simulink model "engine_model"  (R2023b)
settings: Solver=VariableStepAuto  StartTime=0.0  StopTime=10.0  RelTol=1e-3
settings Model: Creator=kirill  LastModifiedBy=kirill
settings DebuggingCC: ModelReferenceExtraNoncontSigs=none

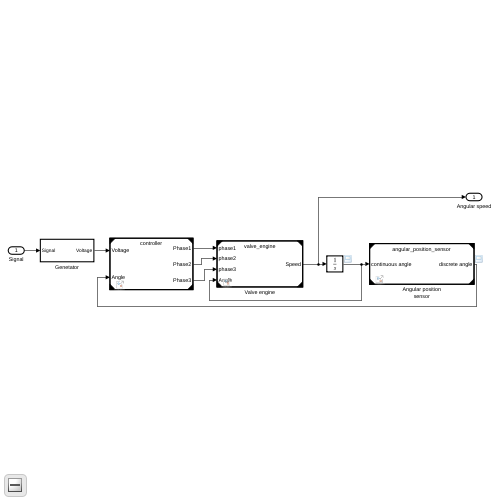
[thumbnail: Simulink's stored preview of the top-level diagram]
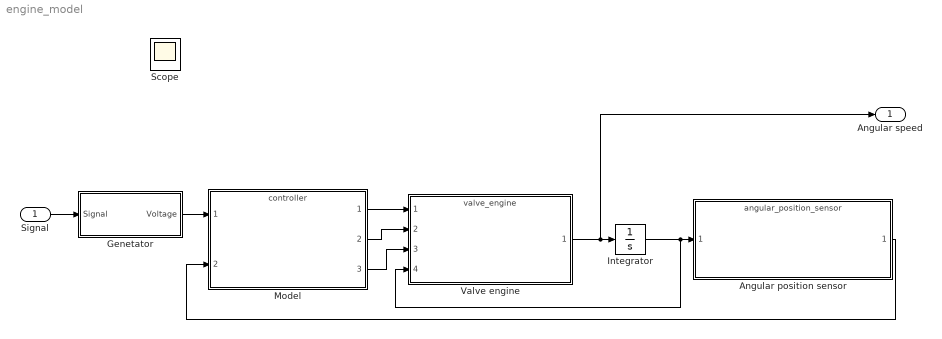
== system engine_model ==
  Signal : Inport
  Angular position sensor : ModelReference  ModelNameDialog=angular_position_sensor.slx  SimulationMode=Normal  ModelReferenceVersion=1.9
  Genetator : Subsystem
  Integrator : Integrator
  Model : ModelReference  ModelNameDialog=controller.slx  SimulationMode=Normal  ModelReferenceVersion=1.9
  Valve engine : ModelReference  ModelNameDialog=valve_engine.slx  SimulationMode=Normal  ModelReferenceVersion=1.25
  Angular speed : Outport
  Scope : Scope
  wires:
  Model/1 -> Valve engine/1
  Model/2 -> Valve engine/2
  Model/3 -> Valve engine/3
  Signal/1 -> Genetator/1(Signal)
  Genetator/1(Voltage) -> Model/1
  Valve engine/1 -> Angular speed/1, Integrator/1
  Integrator/1 -> Valve engine/4, Angular position sensor/1
  Angular position sensor/1 -> Model/2

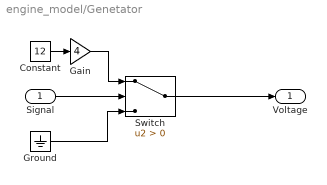
== system engine_model/Genetator ==
  Signal : Inport
  Constant : Constant  Value=12
  Gain : Gain  Gain=4
  Ground : Ground
  Switch : Switch  Criteria=u2 > Threshold  SaturateOnIntegerOverflow=off  InputSameDT=off
  Voltage : Outport
  wires:
  Signal/1 -> Switch/2
  Switch/1 -> Voltage/1
  Ground/1 -> Switch/3
  Constant/1 -> Gain/1
  Gain/1 -> Switch/1
